simulink model "PMSM_SMO_PLL"  (R2023b)
settings: Solver=ode3  StartTime=0.0  StopTime=1  FixedStep=Ts  RelTol=1e-3  EnableMultiTasking=on
InitFcn:
  | R = 2.875;
  | L = 9.8e-3;
  | 
  | Ts=5e-6;
  | 
  | m0 = 2;
  | ksild = 700;
  | A = exp(-R/L*Ts);
  | B = (1-A)/R;
undefined symbols (not defined in the file or in its folder): DiscIntNeverNeededParam
libraries: powerlib_extras x10, spsDCVoltageSourceLib x1, spsGroundLib x1, spsPermanentMagnetSynchronousMachineLib x1, simulink x1, spsThreePhaseVIMeasurementLib x1, spsUniversalBridgeLib x1, sps_lib x1
settings Model: Creator=Administrator  LastModifiedBy=Guoguo
settings SolverCC: AlgebraicLoopSolver=TrustRegion  AutoInsertRateTranBlk=on
settings DataIOCC: LimitDataPoints=on  SaveFormat=Array  SignalLoggingSaveFormat=ModelDataLogs  ReturnWorkspaceOutputs=off
settings OptimizationCC: ExpressionDepthLimit=2147483647  InitFltsAndDblsToZero=on  LifeSpan=inf
settings DebuggingCC: SaveWithParameterizedLinksMsg=none  UnderspecifiedInitializationDetection=Classic  MergeDetectMultiDrivingBlocksExec=none  SolverPrmCheckMsg=warning  FcnCallInpInsideContextMsg=warning  UnconnectedInputMsg=warning  UnconnectedOutputMsg=warning  UnconnectedLineMsg=warning  StateNameClashWarn=warning  SFUnexpectedBacktrackingDiag=warning  SFNoUnconditionalDefaultTransitionDiag=warning  SFExecutionAtInitializationDiag=none  ArithmeticOperatorsInVariantConditions=warning
settings HardwareCC: ProdBitPerPointer=32  ProdBitPerSizeT=32  ProdBitPerPtrDiffT=32  ProdLargestAtomicFloat=None  ProdIntDivRoundTo=Undefined  ProdEndianess=Unspecified  ProdWordSize=32  ProdHWDeviceType=32-bit Generic
settings ModelReferenceCC: EnableRefExpFcnMdlSchedulingChecks=on  PropagateSignalLabelsOutOfModel=off
settings SFSimCC: SimUseLocalCustomCode=off  CustomCodeUndefinedFunction=UseInterfaceOnly
settings RTWCC: RTWUseLocalCustomCode=off  DLArmComputeVersion=19.05
settings CodeAppCC: StateflowObjectComments=on
settings GRTTargetCC: TargetFcnLib=ansi_tfl_tmw.mat  TargetLangStandard=C89/C90 (ANSI)  CombineOutputUpdateFcns=off  GRTInterface=on
settings ConfigComp: CovMetricSettings=dw  CovSaveCumulativeToWorkspaceVar=on  CovSaveSingleToWorkspaceVar=on  CovExternalEMLEnable=off  CovSFcnEnable=off
settings SimscapeCC: SimscapeNormalizeSystem=off

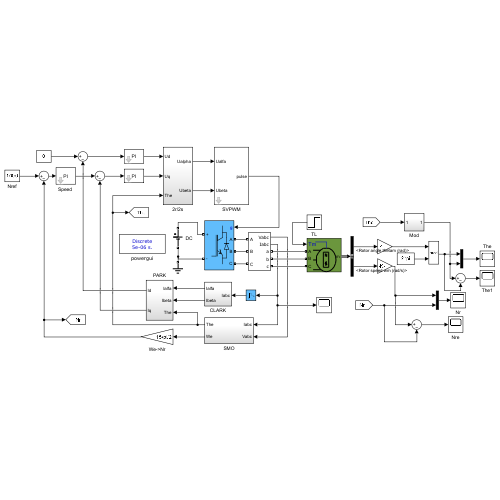
[thumbnail: Simulink's stored preview of the top-level diagram]
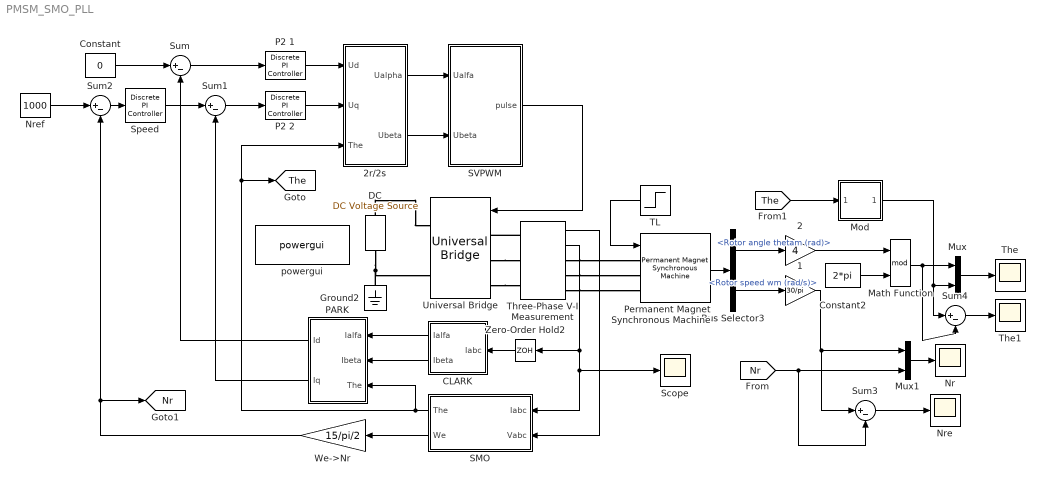
== system PMSM_SMO_PLL ==
  1 : Gain  Gain=30/pi
  2 : Gain  Gain=4
  2r/2s : Subsystem
  Bus Selector3 : BusSelector  OutputSignals=Rotor angle thetam (rad),Rotor speed wm (rad/s)
  CLARK : Subsystem
  Constant : Constant  Value=0
  Constant2 : Constant  Value=2*pi
  "DC " : spsDCVoltageSourceLib/DC Voltage Source  Amplitude=350  Measurements=None
  Ground2 : spsGroundLib/Ground  LConnTagsString=a
  Math Function : Math  Operator=mod  SignedPower=on
  Mod : Subsystem
  Mux : Mux  Inputs=2
  Mux1 : Mux  Inputs=2
  Nr : Scope
  Nre : Scope
  Nref : Constant  Value=1000
  P2 1 : powerlib_extras/Discrete  Control Blocks/Discrete PI Controller  Kp=L*2000  Ki=R*2000  Par_Limits=[350 -350]  Init=0  Ts=Ts
  P2 2 : powerlib_extras/Discrete  Control Blocks/Discrete PI Controller  Kp=L*2000  Ki=R*2000  Par_Limits=[350 -350]  Init=0  Ts=Ts
  PARK : Subsystem
  Permanent Magnet Synchronous Machine : spsPermanentMagnetSynchronousMachineLib/Permanent Magnet Synchronous Machine  NbPhases=3  FluxDistribution=Sinusoidal  RotorType=Salient-pole  MechanicalLoad=Torque Tm  PresetModel=No  ShowDetailedParameters=on  MeasurementBus=off  Resistance=2.875  Inductance=8.5e-3  dqInductances=[8.8e-3 8.8e-3]  La=0.000835  MachineConstant=Flux linkage established by magnets (V.s)  Flux=0.205  VoltageCst=148.7315  TorqueCst=1.23  Flat=120  Mechanical=[1e-3 0 4]  PolePairs=2  InitialConditions=[0,0, 0,0]  InitialConditions5ph=[0 0 0 0 0 0]  RefAngle=Aligned with phase A axis (original Park)  IterativeDiscreteModel=Trapezoidal non iterative  TsBlock=-1  TsPowergui=0
  SMO : Subsystem
  SVPWM : Subsystem  Tag=SVPWM  mask{F=10, Vdc=350}
      mask prompts: F "Chopping　Frequency(KHz)"; Vdc "DC Voltage(V)"
  Scope : Scope
  "Speed " : powerlib_extras/Discrete  Control Blocks/Discrete PI Controller  Kp=0.02  Ki=0.5  Par_Limits=[30 -30]  Init=0  Ts=Ts
  Sum{,1..4} (5 alike) : Sum  Inputs=|+-
  TL : Step  Time=0.5  After=5  SampleTime=0
  The : Scope
  The1 : Scope
  Three-Phase V-I Measurement : spsThreePhaseVIMeasurementLib/Three-Phase V-I Measurement  VoltageMeasurement=phase-to-ground  SetLabelV=off  LabelV=Vabc  Vpu=off  VpuLL=off  CurrentMeasurement=yes  SetLabelI=off  LabelI=Iabc  Ipu=off  Pbase=100e6  Vbase=500e3  OutputType=Complex  PhasorSimulation=off  PSBequivalent=0
  Universal Bridge : spsUniversalBridgeLib/Universal Bridge  Arms=3  SnubberResistance=1e5  SnubberCapacitance=inf  Device=IGBT / Diodes  Ron=1e-3  Lon=0  ForwardVoltages="[  0  0  ]"  ForwardVoltage=0  GTOparameters=[ 10e-6 , 20e-6 ]  IGBTparameters=[ 1e-6 , 2e-6 ]  Measurements=None  Measurements_2=None  converterType=Rectifier
  We->Nr : Gain  Gain=15/pi/2
  Zero-Order Hold2 : ZeroOrderHold  SampleTime=Ts
  powergui : sps_lib/powergui  Priority=1  SimulationMode=Discrete  SampleTime=Ts  frequency=60  Iterations=50  frequencyindice=0  Pbase=100e6  ErrMax=1e-4  UnitsV=kV  UnitsW=MW  buscounter=0  FunctionMessages=off  echomessages=off  EnableUseOfTLC=off  CurrentSourceSwitches=off  DisableSnubberDevices=off  DisableRonSwitches=off  DisableVfSwitches=off  DisplayEquations=off  AutomaticDiscreteSolvers=off  SolverType=Tustin/Backward Euler (TBE)  Interpol=off  ExternalGateDelay=off  methode=off  Ts=0  x0status=blocks  SPID=off  SwTol=0  HookPort=off  NonlinearTolerance=1e-4  nMaxIteration=100  ContinueOnMaxIteration=off  RestoreLinks=warning  ResistiveCurrentMeasurement=off  Frange=[0:2:500]  Ylog=off  Xlog=on  ShowGrid=off  save=off  variable=ZData  structure=0  ZoomFFT=on  StartTime=0.0  cycles=1  DisplayStyle=1  fundamental=60  FreqAxis=off  MaxFrequency=1000  frequencyindicesteady=1  RmsSteady=1  display=off
  tag scope: Nr=global, The=global
  wires:
  SVPWM/1(pulse) -> Universal Bridge/1
  Permanent Magnet Synchronous Machine/1 -> Bus Selector3/1
  P2 1/1 -> 2r/2s/1(Ud)
  P2 2/1 -> 2r/2s/2(Uq)
  Sum/1 -> P2 1/1
  Sum1/1 -> P2 2/1
  "Speed "/1 -> Sum1/1
  Constant/1 -> Sum/1
  Sum2/1 -> "Speed "/1
  Bus Selector3/2 -> 1/1  "<Rotor speed wm (rad/s)>"
  CLARK/2(Ibeta) -> PARK/2(Ibeta)
  CLARK/1(Ialfa) -> PARK/1(Ialfa)
  PARK/1(Id) -> Sum/2
  PARK/2(Iq) -> Sum1/2
  SMO/1(The) -> [The], 2r/2s/3(The), PARK/3(The)
  Zero-Order Hold2/1 -> CLARK/1(Iabc)
  Constant2/1 -> Math Function/2
  2/1 -> Math Function/1
  Bus Selector3/1 -> 2/1  "<Rotor angle thetam (rad)>"
  Mux/1 -> The/1
  Math Function/1 -> Sum4/2, Mux/1
  Mux1/1 -> Nr/1
  1/1 -> Sum3/1, Mux1/1
  SMO/2(We) -> We->Nr/1
  We->Nr/1 -> [Nr], Sum2/2
  TL/1 -> Permanent Magnet Synchronous Machine/1
  2r/2s/2(Ubeta) -> SVPWM/2(Ubeta)
  2r/2s/1(Ualpha) -> SVPWM/1(Ualfa)
  Three-Phase V-I Measurement/2 -> Zero-Order Hold2/1, Scope/1, SMO/1(Iabc)
  Three-Phase V-I Measurement/1 -> SMO/2(Vabc)
  [Nr] -> Sum3/2, Mux1/2
  [The] -> Mod/1(In1)
  Mod/1(Out1) -> Sum4/1, Mux/2
  Sum3/1 -> Nre/1
  Nref/1 -> Sum2/1
  Sum4/1 -> The1/1
  connections:
  "DC "/RConn1 -- Universal Bridge/RConn1
  "DC "/LConn1 -- Ground2/LConn1 -- Universal Bridge/RConn2
  Three-Phase V-I Measurement/LConn1 -- Universal Bridge/LConn1
  Universal Bridge/LConn2 -- Three-Phase V-I Measurement/LConn2
  Universal Bridge/LConn3 -- Three-Phase V-I Measurement/LConn3
  Three-Phase V-I Measurement/RConn1 -- Permanent Magnet Synchronous Machine/LConn1
  Three-Phase V-I Measurement/RConn2 -- Permanent Magnet Synchronous Machine/LConn2
  Three-Phase V-I Measurement/RConn3 -- Permanent Magnet Synchronous Machine/LConn3

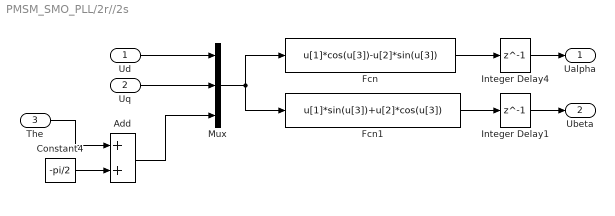
== system PMSM_SMO_PLL/2r//2s ==
  Ud : Inport
  Uq : Inport  Port=2
  The : Inport  Port=3
  Add : Sum
  Constant4 : Constant  Value=-pi/2
  Fcn : Fcn  Expr=u[1]*cos(u[3])-u[2]*sin(u[3])
  Fcn1 : Fcn  Expr=u[1]*sin(u[3])+u[2]*cos(u[3])
  Integer Delay1 : Delay  DelayLength=1  SampleTime=Ts
  Integer Delay4 : Delay  DelayLength=1  SampleTime=Ts
  Mux : Mux  Inputs=3
  Ualpha : Outport
  Ubeta : Outport  Port=2
  wires:
  Ud/1 -> Mux/1
  Uq/1 -> Mux/2
  Mux/1 -> Fcn/1, Fcn1/1
  Fcn/1 -> Integer Delay4/1
  Fcn1/1 -> Integer Delay1/1
  Constant4/1 -> Add/2
  The/1 -> Add/1
  Add/1 -> Mux/3
  Integer Delay4/1 -> Ualpha/1
  Integer Delay1/1 -> Ubeta/1

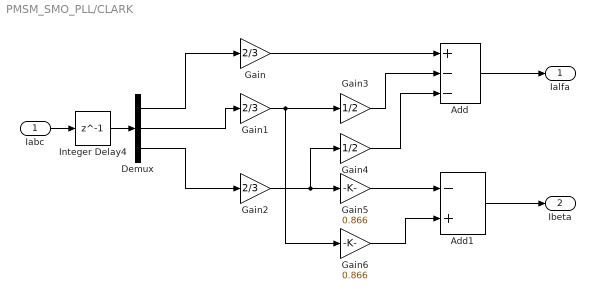
== system PMSM_SMO_PLL/CLARK ==
  Iabc : Inport
  Add : Sum  Inputs=+--
  Add1 : Sum  Inputs=-+
  Demux : Demux  Outputs=3
  Gain : Gain  Gain=2/3
  Gain1 : Gain  Gain=2/3
  Gain2 : Gain  Gain=2/3
  Gain3 : Gain  Gain=1/2
  Gain4 : Gain  Gain=1/2
  Gain5 : Gain  Gain=0.866
  Gain6 : Gain  Gain=0.866
  Integer Delay4 : Delay  DelayLength=1  SampleTime=50e-6
  Ialfa : Outport
  Ibeta : Outport  Port=2
  wires:
  Gain4/1 -> Add/3
  Add/1 -> Ialfa/1
  Add1/1 -> Ibeta/1
  Gain6/1 -> Add1/2
  Gain5/1 -> Add1/1
  Gain2/1 -> Gain4/1, Gain5/1
  Gain3/1 -> Add/2
  Gain1/1 -> Gain6/1, Gain3/1
  Gain/1 -> Add/1
  Demux/1 -> Gain/1
  Demux/2 -> Gain1/1
  Demux/3 -> Gain2/1
  Iabc/1 -> Integer Delay4/1
  Integer Delay4/1 -> Demux/1

== system PMSM_SMO_PLL/Mod ==
  In1 : Inport
  Constant : Constant  Value=2*pi
  Constant1 : Constant  Value=pi/2
  Math Function1 : Math  Operator=mod  SignedPower=on
  Sum4 : Sum  Inputs=-+|
  Out1 : Outport
  wires:
  In1/1 -> Sum4/2
  Constant/1 -> Math Function1/2
  Sum4/1 -> Math Function1/1
  Math Function1/1 -> Out1/1
  Constant1/1 -> Sum4/1

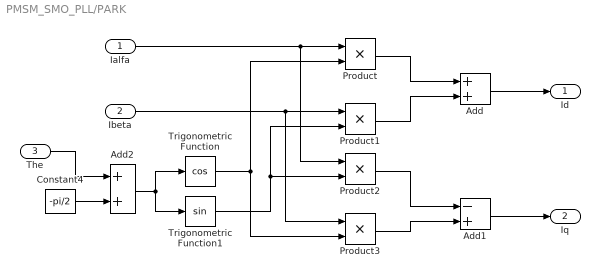
== system PMSM_SMO_PLL/PARK ==
  Ialfa : Inport
  Ibeta : Inport  Port=2
  The : Inport  Port=3
  Add : Sum
  Add1 : Sum  Inputs=-+
  Add2 : Sum
  Constant4 : Constant  Value=-pi/2
  Product{,1..3} (4 alike) : Product  RndMeth=Zero
  Trigonometric Function : Trigonometry  Operator=cos
  Trigonometric Function1 : Trigonometry
  Id : Outport
  Iq : Outport  Port=2
  wires:
  Add1/1 -> Iq/1
  Product3/1 -> Add1/2
  Product2/1 -> Add1/1
  Add/1 -> Id/1
  Product1/1 -> Add/2
  Product/1 -> Add/1
  Trigonometric Function1/1 -> Product2/2, Product1/2
  Trigonometric Function/1 -> Product3/2, Product/2
  Add2/1 -> Trigonometric Function1/1, Trigonometric Function/1
  Ibeta/1 -> Product3/1, Product1/1
  Ialfa/1 -> Product2/1, Product/1
  Constant4/1 -> Add2/2
  The/1 -> Add2/1

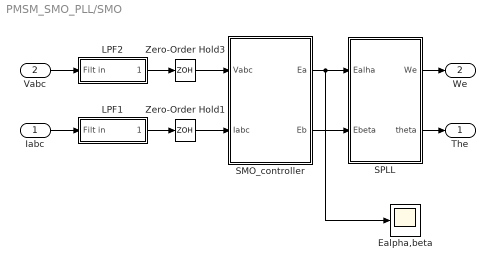
== system PMSM_SMO_PLL/SMO ==
  Iabc : Inport
  Vabc : Inport  Port=2
  Ealpha,beta : Scope
  LPF1 : Subsystem  mask{wcc=3000, Ts=Ts}
      mask prompts: wcc "Control Filter cutoff frequency(Hz):"; Ts "sampling time"
  LPF2 : Subsystem  mask{wcc=3000, Ts=Ts}
      mask prompts: wcc "Control Filter cutoff frequency(Hz):"; Ts "sampling time"
  SMO_controller : Subsystem  mask{Ts=Ts}
  SPLL : Subsystem
  Zero-Order Hold1 : ZeroOrderHold  SampleTime=Ts
  Zero-Order Hold3 : ZeroOrderHold  SampleTime=Ts
  The : Outport
  We : Outport  Port=2
  wires:
  LPF1/1(Filt out) -> Zero-Order Hold1/1
  LPF2/1(Filt out) -> Zero-Order Hold3/1
  Vabc/1 -> LPF2/1(Filt in)
  Zero-Order Hold1/1 -> SMO_controller/2(Iabc)
  Zero-Order Hold3/1 -> SMO_controller/1(Vabc)
  SMO_controller/1(Ea) -> SPLL/1(Ealha), Ealpha,beta/1
  SMO_controller/2(Eb) -> SPLL/2(Ebeta)
  SPLL/1(We) -> We/1
  Iabc/1 -> LPF1/1(Filt in)
  SPLL/2(theta) -> The/1

== system PMSM_SMO_PLL/SVPWM ==
  Ualfa : Inport
  Ubeta : Inport  Port=2
  DC Voltage : Constant  Value=Vdc
  Frequence : Constant  Value=0.001/F
  N1 : Subsystem
  Subsystem : Subsystem
  Subsystem1 : Subsystem
  X.Y.Z : Subsystem
  produce PWM : Subsystem
  pulse : Outport
  wires:
  Ubeta/1 -> X.Y.Z/3(Ubeta), N1/2(Ubeta)
  Subsystem/2(T2) -> Subsystem1/2(T2)
  Subsystem/1(T1) -> Subsystem1/1(T1)
  Ualfa/1 -> N1/1(Ualfa), X.Y.Z/2(Ualfa)
  Subsystem1/3(Tcm3) -> produce PWM/3(Tcm3)
  Subsystem1/2(Tcm2) -> produce PWM/2(Tcm2)
  Subsystem1/1(Tcm1) -> produce PWM/1(Tcm1)
  X.Y.Z/3(Z) -> Subsystem/4(Z)
  X.Y.Z/2(Y) -> Subsystem/3(Y)
  X.Y.Z/1(X) -> Subsystem/2(X)
  N1/1(N) -> Subsystem1/4(N), Subsystem/1(N)
  DC Voltage/1 -> X.Y.Z/4(Udc)
  Frequence/1 -> Subsystem/5(T), Subsystem1/3(T), X.Y.Z/1(T)
  produce PWM/1(pulse) -> pulse/1

== system PMSM_SMO_PLL/SMO/LPF1 ==
  Filt in : Inport
  Demux1 : Demux  Outputs=3
      settings: DisplayOption=none
  LPF1 : powerlib_extras/Discrete  Control Blocks/Discrete 1st-Order Filter  FilterType=Lowpass  Tc=1/(2*pi*wcc)  Ts=Ts  Initialize=off  Vac_Init=[0.8 -25 60]  Vdc_Init=-0.4  PlotResponse=off  param1=[1 500 1]
  LPF2 : powerlib_extras/Discrete  Control Blocks/Discrete 1st-Order Filter  FilterType=Lowpass  Tc=1/(2*pi*wcc)  Ts=Ts  Initialize=off  Vac_Init=[0.8 -25 60]  Vdc_Init=-0.4  PlotResponse=off  param1=[1 500 1]
  LPF3 : powerlib_extras/Discrete  Control Blocks/Discrete 1st-Order Filter  FilterType=Lowpass  Tc=1/(2*pi*wcc)  Ts=Ts  Initialize=off  Vac_Init=[0.8 -25 60]  Vdc_Init=-0.4  PlotResponse=off  param1=[1 4000 1]
  Mux1 : Mux  Inputs=3
  Filt out : Outport
  wires:
  Demux1/1 -> LPF1/1
  LPF1/1 -> Mux1/1
  Demux1/2 -> LPF2/1
  LPF2/1 -> Mux1/2
  Filt in/1 -> Demux1/1
  Mux1/1 -> Filt out/1
  Demux1/3 -> LPF3/1
  LPF3/1 -> Mux1/3

== system PMSM_SMO_PLL/SMO/LPF2 ==
  Filt in : Inport
  Demux1 : Demux  Outputs=3
      settings: DisplayOption=none
  LPF1 : powerlib_extras/Discrete  Control Blocks/Discrete 1st-Order Filter  FilterType=Lowpass  Tc=1/(2*pi*wcc)  Ts=Ts  Initialize=off  Vac_Init=[0.8 -25 60]  Vdc_Init=-0.4  PlotResponse=off  param1=[1 500 1]
  LPF2 : powerlib_extras/Discrete  Control Blocks/Discrete 1st-Order Filter  FilterType=Lowpass  Tc=1/(2*pi*wcc)  Ts=Ts  Initialize=off  Vac_Init=[0.8 -25 60]  Vdc_Init=-0.4  PlotResponse=off  param1=[1 500 1]
  LPF3 : powerlib_extras/Discrete  Control Blocks/Discrete 1st-Order Filter  FilterType=Lowpass  Tc=1/(2*pi*wcc)  Ts=Ts  Initialize=off  Vac_Init=[0.8 -25 60]  Vdc_Init=-0.4  PlotResponse=off  param1=[1 4000 1]
  Mux1 : Mux  Inputs=3
  Filt out : Outport
  wires:
  LPF3/1 -> Mux1/3
  Demux1/3 -> LPF3/1
  Mux1/1 -> Filt out/1
  Filt in/1 -> Demux1/1
  LPF2/1 -> Mux1/2
  Demux1/2 -> LPF2/1
  LPF1/1 -> Mux1/1
  Demux1/1 -> LPF1/1

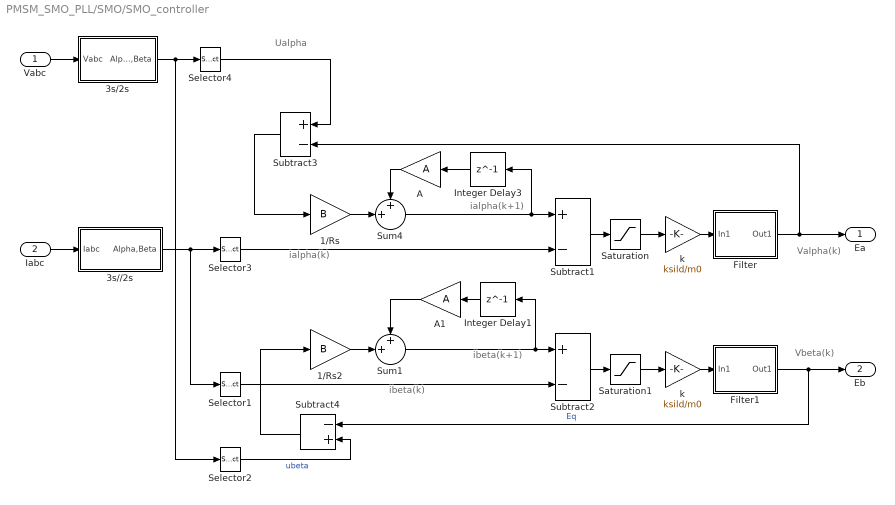
== system PMSM_SMO_PLL/SMO/SMO_controller ==
  note: Vbeta(k)
  note: ibeta(k+1)
  note: ibeta(k)
  note: ialpha(k+1)
  note: Valpha(k)
  note: ialpha(k)
  note: Ualpha
  Vabc : Inport
  Iabc : Inport  Port=2
  1/Rs : Gain  Gain=B
  1/Rs2 : Gain  Gain=B
  3s//2s : Subsystem
  3s/2s : Subsystem
  A : Gain  Gain=A
  A1 : Gain  Gain=A
  Filter : Subsystem  mask{a=0.97}
  Filter1 : Subsystem  mask{a=0.97}
  Integer Delay1 : Delay  DelayLength=1  SampleTime=Ts
  Integer Delay3 : Delay  DelayLength=1  SampleTime=Ts
  Saturation : Saturate  UpperLimit=m0  LowerLimit=-m0
  Saturation1 : Saturate  UpperLimit=m0  LowerLimit=-m0
  Selector1 : Selector  InputPortWidth=2  IndexOptions=Index vector (dialog)  Indices=[2 ]  OutputSizes=1
  Selector2 : Selector  InputPortWidth=2  IndexOptions=Index vector (dialog)  Indices=[2 ]  OutputSizes=1
  Selector3 : Selector  InputPortWidth=2  IndexOptions=Index vector (dialog)  Indices=[1 ]  OutputSizes=1
  Selector4 : Selector  InputPortWidth=2  IndexOptions=Index vector (dialog)  Indices=[1 ]  OutputSizes=1
  Subtract1 : Sum  Inputs=+-
  Subtract2 : Sum  Inputs=+-
  Subtract3 : Sum  Inputs=+-
  Subtract4 : Sum  Inputs=-+
  Sum1 : Sum  Inputs=++|
  Sum4 : Sum  Inputs=++|
  k : Gain  Gain=ksild/m0
  "k " : Gain  Gain=ksild/m0
  Ea : Outport
  Eb : Outport  Port=2
  wires:
  3s//2s/1(Alpha,Beta) -> Selector1/1, Selector3/1
  Filter/1(Out1) -> Subtract3/2, Ea/1
  Saturation/1 -> "k "/1
  Integer Delay3/1 -> A/1
  Sum4/1 -> Integer Delay3/1, Subtract1/1
  Subtract1/1 -> Saturation/1
  "k "/1 -> Filter/1(In1)
  Subtract3/1 -> 1/Rs/1
  1/Rs/1 -> Sum4/2
  A/1 -> Sum4/1
  Selector3/1 -> Subtract1/2
  Saturation1/1 -> k/1
  Integer Delay1/1 -> A1/1
  Sum1/1 -> Integer Delay1/1, Subtract2/1
  Subtract2/1 -> Saturation1/1
  k/1 -> Filter1/1(In1)
  Subtract4/1 -> 1/Rs2/1
  1/Rs2/1 -> Sum1/2
  A1/1 -> Sum1/1
  Selector1/1 -> Subtract2/2
  Vabc/1 -> 3s/2s/1(Vabc)
  Iabc/1 -> 3s//2s/1(Iabc)
  3s/2s/1(Alpha,Beta) -> Selector4/1, Selector2/1
  Selector4/1 -> Subtract3/1
  Filter1/1(Out1) -> Subtract4/1, Eb/1  "Eq"
  Selector2/1 -> Subtract4/2  "ubeta"

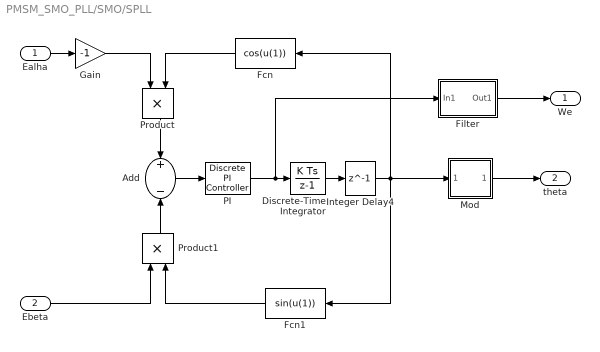
== system PMSM_SMO_PLL/SMO/SPLL ==
  Ealha : Inport
  Ebeta : Inport  Port=2
  Add : Sum  Inputs=+-
  Discrete-Time Integrator : DiscreteIntegrator  SampleTime=Ts  ICPrevOutput=DiscIntNeverNeededParam  ICPrevScaledInput=DiscIntNeverNeededParam
  Fcn : Fcn  Expr=cos(u(1))
  Fcn1 : Fcn  Expr=sin(u(1))
  Filter : Subsystem  mask{a=0.99}
  Gain : Gain  Gain=-1
  Integer Delay4 : Delay  DelayLength=1  SampleTime=Ts
  Mod : Subsystem
  PI : powerlib_extras/Discrete  Control Blocks/Discrete PI Controller  Kp=13.8  Ki=144.3  Par_Limits="[5000  -5000]"  Init=0  Ts=Ts
  Product : Product  RndMeth=Zero
  Product1 : Product  RndMeth=Zero
  We : Outport
  theta : Outport  Port=2
  wires:
  Discrete-Time Integrator/1 -> Integer Delay4/1
  Ebeta/1 -> Product1/1
  Add/1 -> PI/1
  Product/1 -> Add/1
  Fcn/1 -> Product/2
  Product1/1 -> Add/2
  Fcn1/1 -> Product1/2
  Ealha/1 -> Gain/1
  Gain/1 -> Product/1
  PI/1 -> Discrete-Time Integrator/1, Filter/1(In1)
  Integer Delay4/1 -> Fcn1/1, Mod/1(In1), Fcn/1
  Filter/1(Out1) -> We/1
  Mod/1(Out1) -> theta/1

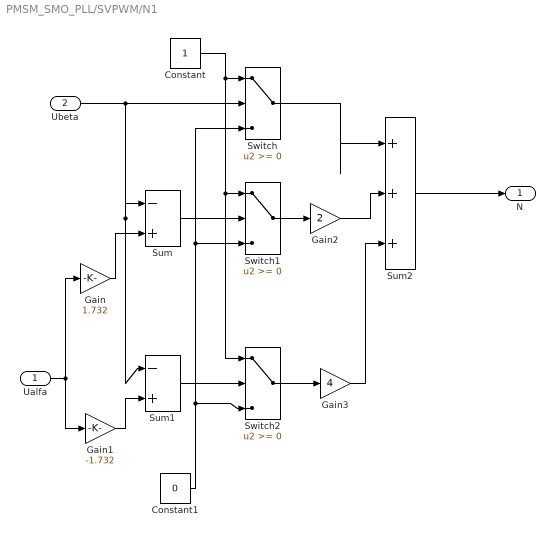
== system PMSM_SMO_PLL/SVPWM/N1 ==
  Ualfa : Inport
  Ubeta : Inport  Port=2
  Constant : Constant
  Constant1 : Constant  Value=0
  Gain : Gain  Gain=1.732
  Gain1 : Gain  Gain=-1.732
  Gain2 : Gain  Gain=2
  Gain3 : Gain  Gain=4
  Sum : Sum  Inputs=|-+
  Sum1 : Sum  Inputs=|-+
  Sum2 : Sum  Inputs=|+++
  Switch : Switch  SaturateOnIntegerOverflow=off  InputSameDT=off
  Switch1 : Switch  SaturateOnIntegerOverflow=off  InputSameDT=off
  Switch2 : Switch  SaturateOnIntegerOverflow=off  InputSameDT=off
  N : Outport
  wires:
  Sum2/1 -> N/1
  Gain3/1 -> Sum2/3
  Switch/1 -> Sum2/1
  Gain2/1 -> Sum2/2
  Switch2/1 -> Gain3/1
  Switch1/1 -> Gain2/1
  Constant1/1 -> Switch2/3, Switch1/3, Switch/3
  Gain1/1 -> Sum1/2
  Sum1/1 -> Switch2/2
  Sum/1 -> Switch1/2
  Gain/1 -> Sum/2
  Ualfa/1 -> Gain/1, Gain1/1
  Constant/1 -> Switch1/1, Switch2/1, Switch/1
  Ubeta/1 -> Sum1/1, Sum/1, Switch/2

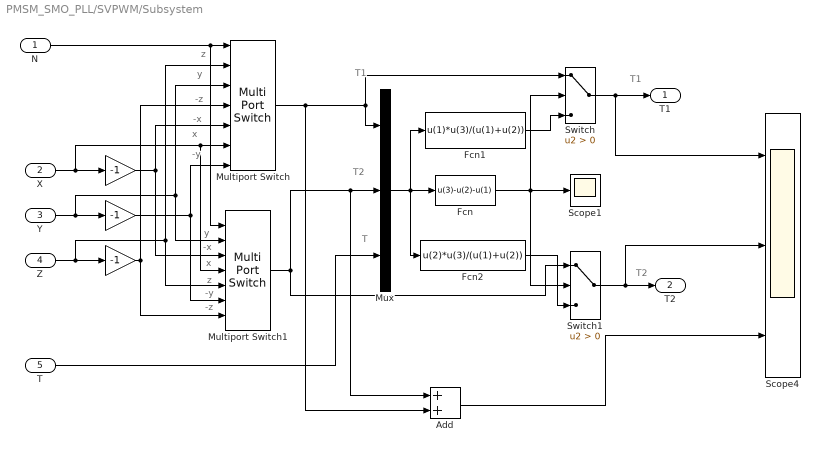
== system PMSM_SMO_PLL/SVPWM/Subsystem ==
  note: T2
  note: T1
  note: T
  note: T2
  note: T1
  note: -z
  note: -y
  note: z
  note: x
  note: -x
  note: y
  note: -y
  note: x
  note: -x
  note: -z
  note: y
  note: z
  N : Inport
  X : Inport  Port=2
  Y : Inport  Port=3
  Z : Inport  Port=4
  T : Inport  Port=5
  " " : Gain  Gain=-1
  "  " : Gain  Gain=-1
  "    " : Gain  Gain=-1
  Add : Sum
  Fcn : Fcn  Expr=u(3)-u(2)-u(1)
  Fcn1 : Fcn  Expr=u(1)*u(3)/(u(1)+u(2))
  Fcn2 : Fcn  Expr=u(2)*u(3)/(u(1)+u(2))
  Multiport Switch : MultiPortSwitch  Inputs=6  DiagnosticForDefault=None  SaturateOnIntegerOverflow=off  InputSameDT=off
  Multiport Switch1 : MultiPortSwitch  Inputs=6  DiagnosticForDefault=None  SaturateOnIntegerOverflow=off  InputSameDT=off
  Mux : Mux  Inputs=3
  Scope1 : Scope
  Scope4 : Scope  NumInputPorts=3
  Switch : Switch  Criteria=u2 > Threshold  SaturateOnIntegerOverflow=off  InputSameDT=off
  Switch1 : Switch  Criteria=u2 > Threshold  SaturateOnIntegerOverflow=off  InputSameDT=off
  T1 : Outport
  T2 : Outport  Port=2
  wires:
  Add/1 -> Scope4/3
  Switch1/1 -> Scope4/2, T2/1
  Switch/1 -> Scope4/1, T1/1
  Fcn2/1 -> Switch1/3
  Fcn1/1 -> Switch/3
  Mux/1 -> Fcn2/1, Fcn1/1, Fcn/1
  T/1 -> Mux/3
  Multiport Switch/1 -> Add/2, Switch/1, Mux/1
  " "/1 -> Multiport Switch1/3, Multiport Switch/5
  "  "/1 -> Multiport Switch1/6, Multiport Switch/7
  "    "/1 -> Multiport Switch/4, Multiport Switch1/7
  Z/1 -> "    "/1, Multiport Switch/2, Multiport Switch1/5
  Y/1 -> "  "/1, Multiport Switch/3, Multiport Switch1/2
  X/1 -> " "/1, Multiport Switch/6, Multiport Switch1/4
  N/1 -> Multiport Switch/1, Multiport Switch1/1
  Fcn/1 -> Scope1/1, Switch1/2, Switch/2
  Multiport Switch1/1 -> Add/1, Mux/2, Switch1/1

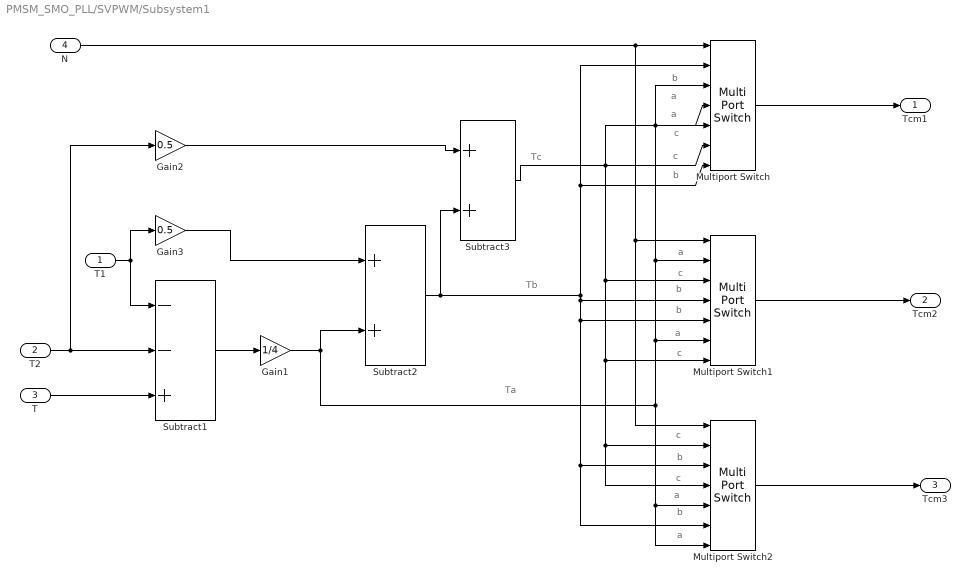
== system PMSM_SMO_PLL/SVPWM/Subsystem1 ==
  note: a
  note: b
  note: a
  note: c
  note: b
  note: c
  note: c
  note: a
  note: b
  note: b
  note: c
  note: a
  note: b
  note: c
  note: c
  note: a
  note: a
  note: b
  note: Tc
  note: Tb
  note: Ta
  T1 : Inport
  T2 : Inport  Port=2
  T : Inport  Port=3
  N : Inport  Port=4
  Gain1 : Gain  Gain=1/4
  Gain2 : Gain  Gain=0.5
  Gain3 : Gain  Gain=0.5
  Multiport Switch : MultiPortSwitch  Inputs=6  DiagnosticForDefault=None  SaturateOnIntegerOverflow=off  InputSameDT=off
  Multiport Switch1 : MultiPortSwitch  Inputs=6  DiagnosticForDefault=None  SaturateOnIntegerOverflow=off  InputSameDT=off
  Multiport Switch2 : MultiPortSwitch  Inputs=6  DiagnosticForDefault=None  SaturateOnIntegerOverflow=off  InputSameDT=off
  Subtract1 : Sum  Inputs=--+
  Subtract2 : Sum
  Subtract3 : Sum
  Tcm1 : Outport
  Tcm2 : Outport  Port=2
  Tcm3 : Outport  Port=3
  wires:
  Subtract3/1 -> Multiport Switch2/4, Multiport Switch2/2, Multiport Switch1/7, Multiport Switch1/3, Multiport Switch/6, Multiport Switch/5
  N/1 -> Multiport Switch1/1, Multiport Switch2/1, Multiport Switch/1
  Gain2/1 -> Subtract3/1
  Subtract2/1 -> Multiport Switch2/6, Multiport Switch2/3, Multiport Switch1/5, Multiport Switch1/4, Multiport Switch/7, Multiport Switch/2, Subtract3/2
  Gain1/1 -> Subtract2/2, Multiport Switch1/6, Multiport Switch1/2, Multiport Switch/4, Multiport Switch/3, Multiport Switch2/7, Multiport Switch2/5
  Subtract1/1 -> Gain1/1
  Gain3/1 -> Subtract2/1
  T1/1 -> Subtract1/1, Gain3/1
  T/1 -> Subtract1/3
  T2/1 -> Subtract1/2, Gain2/1
  Multiport Switch/1 -> Tcm1/1
  Multiport Switch1/1 -> Tcm2/1
  Multiport Switch2/1 -> Tcm3/1

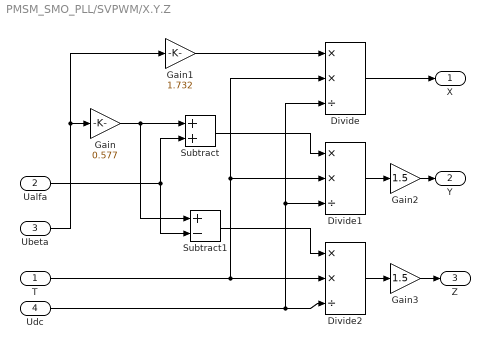
== system PMSM_SMO_PLL/SVPWM/X.Y.Z ==
  T : Inport
  Ualfa : Inport  Port=2
  Ubeta : Inport  Port=3
  Udc : Inport  Port=4
  Divide : Product  Inputs=**/
  Divide1 : Product  Inputs=**/
  Divide2 : Product  Inputs=**/
  Gain : Gain  Gain=0.577
  Gain1 : Gain  Gain=1.732
  Gain2 : Gain  Gain=1.5
  Gain3 : Gain  Gain=1.5
  Subtract : Sum
  Subtract1 : Sum  Inputs=+-
  X : Outport
  Y : Outport  Port=2
  Z : Outport  Port=3
  wires:
  Ubeta/1 -> Gain/1, Gain1/1
  Gain3/1 -> Z/1
  Gain2/1 -> Y/1
  Divide2/1 -> Gain3/1
  Divide1/1 -> Gain2/1
  Divide/1 -> X/1
  Subtract1/1 -> Divide2/1
  Subtract/1 -> Divide1/1
  Ualfa/1 -> Subtract/2, Subtract1/2
  Udc/1 -> Divide/3, Divide1/3, Divide2/3
  T/1 -> Divide/2, Divide1/2, Divide2/2
  Gain1/1 -> Divide/1
  Gain/1 -> Subtract1/1, Subtract/1

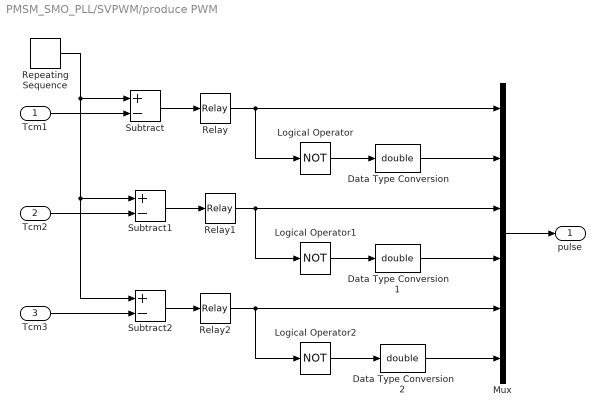
== system PMSM_SMO_PLL/SVPWM/produce PWM ==
  Tcm1 : Inport
  Tcm2 : Inport  Port=2
  Tcm3 : Inport  Port=3
  Data Type Conversion : DataTypeConversion  OutDataTypeStr=double  SaturateOnIntegerOverflow=off  RndMeth=Floor
  Data Type Conversion1 : DataTypeConversion  OutDataTypeStr=double  SaturateOnIntegerOverflow=off  RndMeth=Floor
  Data Type Conversion2 : DataTypeConversion  OutDataTypeStr=double  SaturateOnIntegerOverflow=off  RndMeth=Floor
  Logical Operator : Logic  Operator=NOT  AllPortsSameDT=off
  Logical Operator1 : Logic  Operator=NOT  AllPortsSameDT=off
  Logical Operator2 : Logic  Operator=NOT  AllPortsSameDT=off
  Mux : Mux  Inputs=6
  Relay : Relay
  Relay1 : Relay
  Relay2 : Relay
  Repeating Sequence : simulink/Sources/Repeating Sequence  rep_seq_t=[0 0.001/F 0.002/F]  rep_seq_y=[0 0.001/F 0]
  Subtract : Sum  Inputs=+-
  Subtract1 : Sum  Inputs=+-
  Subtract2 : Sum  Inputs=+-
  pulse : Outport
  wires:
  Data Type Conversion2/1 -> Mux/6
  Data Type Conversion1/1 -> Mux/4
  Data Type Conversion/1 -> Mux/2
  Mux/1 -> pulse/1
  Relay2/1 -> Mux/5, Logical Operator2/1
  Relay1/1 -> Mux/3, Logical Operator1/1
  Relay/1 -> Mux/1, Logical Operator/1
  Logical Operator/1 -> Data Type Conversion/1
  Logical Operator2/1 -> Data Type Conversion2/1
  Logical Operator1/1 -> Data Type Conversion1/1
  Tcm3/1 -> Subtract2/2
  Tcm2/1 -> Subtract1/2
  Tcm1/1 -> Subtract/2
  Repeating Sequence/1 -> Subtract1/1, Subtract2/1, Subtract/1
  Subtract2/1 -> Relay2/1
  Subtract1/1 -> Relay1/1
  Subtract/1 -> Relay/1

== system PMSM_SMO_PLL/SMO/SMO_controller/3s////2s ==
  Iabc : Inport
  Alpha : Fcn  Expr=2/3*(u(1)-1/2*(u(2)+u(3)))
  Beta : Fcn  Expr=2/3*sqrt(3)/2*(u(2)-u(3))
  Mux : Mux  Inputs=2
  Alpha,Beta : Outport
  wires:
  Mux/1 -> Alpha,Beta/1
  Beta/1 -> Mux/2
  Alpha/1 -> Mux/1
  Iabc/1 -> Beta/1, Alpha/1

== system PMSM_SMO_PLL/SMO/SMO_controller/3s//2s ==
  Vabc : Inport
  Alpha : Fcn  Expr=2/3*(u(1)-1/2*(u(2)+u(3)))
  Beta : Fcn  Expr=2/3*sqrt(3)/2*(u(2)-u(3))
  Mux : Mux  Inputs=2
  Alpha,Beta : Outport
  wires:
  Vabc/1 -> Alpha/1, Beta/1
  Alpha/1 -> Mux/1
  Beta/1 -> Mux/2
  Mux/1 -> Alpha,Beta/1

== system PMSM_SMO_PLL/SMO/SMO_controller/Filter ==
  In1 : Inport
  1/Ld1 : Gain  Gain=a
  1/Ld4 : Gain  Gain=1-a  SampleTime=Ts
  Integer Delay5 : Delay  DelayLength=1  SampleTime=Ts
  Subtract3 : Sum
  Out1 : Outport
  wires:
  In1/1 -> 1/Ld4/1
  1/Ld1/1 -> Subtract3/2
  1/Ld4/1 -> Subtract3/1
  Integer Delay5/1 -> 1/Ld1/1
  Subtract3/1 -> Out1/1, Integer Delay5/1

== system PMSM_SMO_PLL/SMO/SMO_controller/Filter1 ==
  In1 : Inport
  1/Ld1 : Gain  Gain=a
  1/Ld4 : Gain  Gain=1-a  SampleTime=Ts
  Integer Delay5 : Delay  DelayLength=1  SampleTime=Ts
  Subtract3 : Sum
  Out1 : Outport
  wires:
  In1/1 -> 1/Ld4/1
  1/Ld1/1 -> Subtract3/2
  1/Ld4/1 -> Subtract3/1
  Integer Delay5/1 -> 1/Ld1/1
  Subtract3/1 -> Out1/1, Integer Delay5/1

== system PMSM_SMO_PLL/SMO/SPLL/Filter ==
  In1 : Inport
  1/Ld1 : Gain  Gain=a
  1/Ld4 : Gain  Gain=1-a  SampleTime=Ts
  Integer Delay5 : Delay  DelayLength=1  SampleTime=Ts
  Subtract3 : Sum
  Out1 : Outport
  wires:
  In1/1 -> 1/Ld4/1
  1/Ld1/1 -> Subtract3/2
  1/Ld4/1 -> Subtract3/1
  Integer Delay5/1 -> 1/Ld1/1
  Subtract3/1 -> Out1/1, Integer Delay5/1

== system PMSM_SMO_PLL/SMO/SPLL/Mod ==
  In1 : Inport
  Constant : Constant  Value=2*pi
  Constant1 : Constant  Value=pi/2
  Math Function1 : Math  Operator=mod  SignedPower=on
  Sum4 : Sum  Inputs=++|
  Out1 : Outport
  wires:
  In1/1 -> Sum4/2
  Constant/1 -> Math Function1/2
  Sum4/1 -> Math Function1/1
  Math Function1/1 -> Out1/1
  Constant1/1 -> Sum4/1
